simulink model "ident_sim"  (R2015b)
settings: Solver=VariableStepAuto  StartTime=0.0  StopTime=10.0  RelTol=1e-3
values from neighbouring files (symbols this model uses):
  A = [1 -3.92385672485 5.78086735469 -3.78994566567 0.932935089992]    [nyttforsok.mat]    (also in simuleradData.mat)
  A_h = [	0, 1, 0, 0; 	-K_lin/J_1, -(K_m*N)^2/(R_m*J_1), K_lin/J_1, 0; 	0, 0, 0, 1; 	K_lin/J_2, 0, -K_lin/J_2, 0]    [labassignment_dat.m]    (also in nyttforsok.mat = [0 -7000 0 2479.16666667 1 -52.8359980942 0 0 0 7000 0 -2479; simuleradData.mat = [0 -7000 0 2479.16666667 1 -52.8359980942 0 0 0 7000 0 -2479)
  B = [0 0 0.000410578864918 -0.000456577532516]    [nyttforsok.mat]    (also in simuleradData.mat)
  B_h = [	0; 	(N*K_m)/(R_m*J_1); 	0; 	0]    [labassignment_dat.m]    (also in nyttforsok.mat = [0 98.3983873923 0 0]; simuleradData.mat = [0 98.3983873923 0 0])
  dt = 0.001    [nyttforsok.mat]    (also in simuleradData.mat)
settings Model: Creator=rickardandersson  LastModifiedBy=rickardandersson

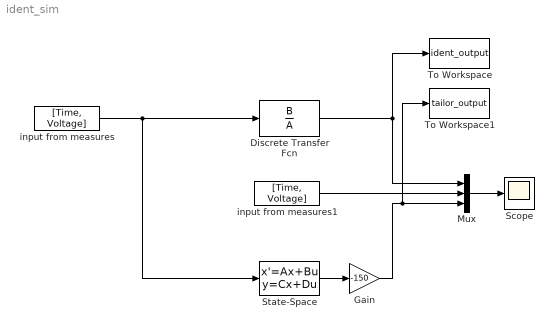
== system ident_sim ==
  Discrete Transfer Fcn : DiscreteTransferFcn  Numerator=B  Denominator=A
  Gain : Gain  Gain=-150
  Mux : Mux  Inputs=3
  Scope : Scope
  State-Space : StateSpace  A=A_h  B=B_h  C=[1 0 0 0]  D=[0]  X0=0
  To Workspace : ToWorkspace  VariableName=ident_output  SaveFormat=Timeseries  SampleTime=-1
  To Workspace1 : ToWorkspace  VariableName=tailor_output  SaveFormat=Timeseries  SampleTime=-1
  input from measures : FromWorkspace  VariableName=[Time, Voltage]  SampleTime=dt
  input from measures1 : FromWorkspace  VariableName=[Time, Voltage]  SampleTime=dt
  wires:
  input from measures/1 -> State-Space/1, Discrete Transfer Fcn/1
  Mux/1 -> Scope/1
  Discrete Transfer Fcn/1 -> Mux/1, To Workspace/1
  input from measures1/1 -> Mux/2
  State-Space/1 -> Gain/1
  Gain/1 -> To Workspace1/1, Mux/3
